simulink model "cmtdtool_sampleharness"  (Simulink 7.1)
settings: Solver=FixedStepDiscrete  StartTime=0.0  StopTime=10.0  FixedStep=0.01  RelTol=1e-3
undefined symbols (not defined in the file or in its folder): DiscIntNeverNeededParam, sigbuilder_block
libraries: simulink x2
settings Model: SldvGeneratedHarnessModel=TestUnitModel=cmtdtool_samplemode|  Creator=The MathWorks Inc.  LastModifiedBy=itoy  CovMetricSettings=dcmoe  CovHTMLOptions=-aTS=1 -bRG=1 -bTC=0 -hTR=0 -nFC=0 -scm=1 -bcm=1 -xEv=0  covSaveCumulativeToWorkspaceVar=off  CovSaveSingleToWorkspaceVar=off  CovModelRefEnable=off
settings OptimizationCC: ConditionallyExecuteInputs=off  InlineParams=on  InlineInvariantSignals=on
settings DebuggingCC: SaveWithParameterizedLinksMsg=none  SignalResolutionControl=TryResolveAllWithWarning  InheritedTsInSrcMsg=none
settings GRTTargetCC: TargetFcnLib=ansi_tfl_tmw.mat  CPPClassGenCompliant=off
settings ConfigComp: Description=Design Verifier Custom Configuration Component  DVMaxProcessTime=60  DVDisplayUnsatisfiableObjectives=on  DVAutomaticStubbing=off  DVMakeOutputFilesUnique=off  DVParameters=on  DVModelCoverageObjectives=MCDC  DVMaxTestCaseSteps=500  DVTestSuiteOptimization=CombinedObjectives  DVAssertions=EnableAll  DVProofAssumptions=EnableAll  DVProvingStrategy=FindViolation  DVSaveHarnessModel=on  DVSaveReport=on

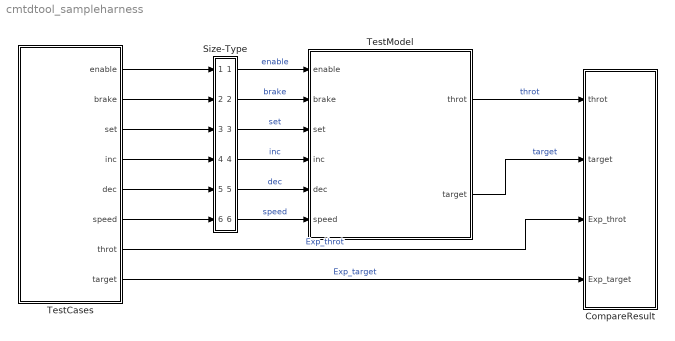
== system cmtdtool_sampleharness ==
  CompareResult : Subsystem  DisableCoverage=on
  Size-Type : Subsystem
  TestCases : Subsystem  Tag=STV Subsys  LoadFcn=sigbuilder_block('load',[49.5 50.25 519.75 399.75 ]);  StartFcn=sigbuilder_block('start');  StopFcn=sigbuilder_block('stop');  ClipboardFcn=sigbuilder_block('clipboard');  mask(Sigbuilder block){}
      mask init:
      | if ~strcmp(get_param(bdroot(gcb),'SimulationStatus'),'stopped') tuvar = sigbuilder_block('maskInit'); end
      settings: CopyFcn=sigbuilder_block('copy');  DeleteFcn=sigbuilder_block('delete');  ModelCloseFcn=sigbuilder_block('modelClose');  PreSaveFcn=sigbuilder_block('preSave');  NameChangeFcn=sigbuilder_block('namechange');  OpenFcn=sigbuilder_block('open');  CloseFcn=sigbuilder_block('close');
      mask Display: plot(0,0,100,100,[10,10,40,40,10],[80,20,20,80,80],[40,10],[50,50], [40,27,10],[65,72,56],[40,25,25,10],[28,28,43,43]);
  TestModel : Subsystem
  wires:
  Size-Type/1(Out1) -> TestModel/1(enable)  "enable"
  Size-Type/2(Out2) -> TestModel/2(brake)  "brake"
  Size-Type/3(Out3) -> TestModel/3(set)  "set"
  Size-Type/4(Out4) -> TestModel/4(inc)  "inc"
  Size-Type/5(Out5) -> TestModel/5(dec)  "dec"
  Size-Type/6(Out6) -> TestModel/6(speed)  "speed"
  TestCases/1(enable) -> Size-Type/1(In1)
  TestCases/2(brake) -> Size-Type/2(In2)
  TestCases/3(set) -> Size-Type/3(In3)
  TestCases/4(inc) -> Size-Type/4(In4)
  TestCases/5(dec) -> Size-Type/5(In5)
  TestCases/6(speed) -> Size-Type/6(In6)
  TestModel/1(throt) -> CompareResult/1(throt)  "throt"
  TestCases/7(throt) -> CompareResult/3(Exp_throt)  "Exp_throt"
  TestModel/2(target) -> CompareResult/2(target)  "target"
  TestCases/8(target) -> CompareResult/4(Exp_target)  "Exp_target"

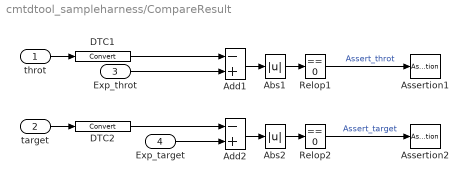
== system cmtdtool_sampleharness/CompareResult ==
  throt : Inport
  target : Inport  Port=2
  Exp_throt : Inport  Port=3
  Exp_target : Inport  Port=4
  Abs1 : Abs  SaturateOnIntegerOverflow=on
  Abs2 : Abs  SaturateOnIntegerOverflow=on
  Add1 : Sum  Inputs=-+  AccumDataTypeStr=double  OutDataTypeStr=double  SaturateOnIntegerOverflow=on  InputSameDT=on
  Add2 : Sum  Inputs=-+  AccumDataTypeStr=double  OutDataTypeStr=double  SaturateOnIntegerOverflow=on  InputSameDT=on
  Assertion1 : Assertion  Enabled=on  StopWhenAssertionFail=off
  Assertion2 : Assertion  Enabled=on  StopWhenAssertionFail=off
  DTC1 : DataTypeConversion
  DTC2 : DataTypeConversion
  Relop1 : simulink/Logic and Bit Operations/Compare To Constant  SystemSampleTime=-1  relop===  const=0  LogicOutDataTypeMode=uint8
  Relop2 : simulink/Logic and Bit Operations/Compare To Constant  SystemSampleTime=-1  relop===  const=0  LogicOutDataTypeMode=uint8
  wires:
  DTC1/1 -> Add1/1
  Add1/1 -> Abs1/1
  Abs1/1 -> Relop1/1
  Relop1/1 -> Assertion1/1  "Assert_throt"
  DTC2/1 -> Add2/1
  Add2/1 -> Abs2/1
  Abs2/1 -> Relop2/1
  Relop2/1 -> Assertion2/1  "Assert_target"
  throt/1 -> DTC1/1
  Exp_throt/1 -> Add1/2
  target/1 -> DTC2/1
  Exp_target/1 -> Add2/2

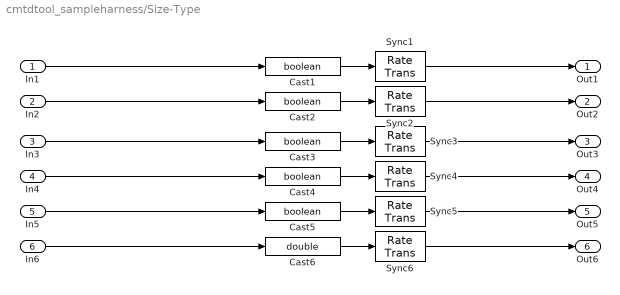
== system cmtdtool_sampleharness/Size-Type ==
  In1 : Inport
  In2 : Inport  Port=2
  In3 : Inport  Port=3
  In4 : Inport  Port=4
  In5 : Inport  Port=5
  In6 : Inport  Port=6
  Cast{1..5} (5 alike) : DataTypeConversion  OutDataTypeStr=boolean  SaturateOnIntegerOverflow=on  RndMeth=Zero
  Cast6 : DataTypeConversion  OutDataTypeStr=double  SaturateOnIntegerOverflow=on  RndMeth=Zero
  Sync{1..6} (6 alike) : RateTransition  OutPortSampleTime=[0.01,0]
  Out1 : Outport
  Out2 : Outport  Port=2
  Out3 : Outport  Port=3
  Out4 : Outport  Port=4
  Out5 : Outport  Port=5
  Out6 : Outport  Port=6
  wires:
  In1/1 -> Cast1/1
  Cast1/1 -> Sync1/1
  Sync1/1 -> Out1/1
  In2/1 -> Cast2/1
  Cast2/1 -> Sync2/1
  Sync2/1 -> Out2/1
  In3/1 -> Cast3/1
  Cast3/1 -> Sync3/1
  Sync3/1 -> Out3/1
  In4/1 -> Cast4/1
  Cast4/1 -> Sync4/1
  Sync4/1 -> Out4/1
  In5/1 -> Cast5/1
  Cast5/1 -> Sync5/1
  Sync5/1 -> Out5/1
  In6/1 -> Cast6/1
  Cast6/1 -> Sync6/1
  Sync6/1 -> Out6/1

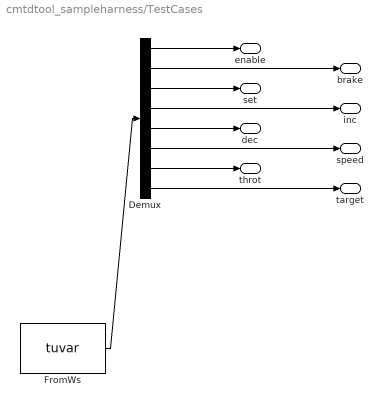
== system cmtdtool_sampleharness/TestCases ==
  Demux : Demux  Tag=STV Demux  Outputs=8
  FromWs : FromWorkspace  Tag=STV FromWs  VariableName=tuvar  SampleTime=0  SigBuilderData=DataTag0  VnvData=DataTag1
      SigBuilderData=|
      | channels(1).label = 'enable'
      | channels(1).allXData = {[0 0.01 0.02 0.03 0.04 0.05 0.06 0.07 0.08 0.09 0.1 0.11], [0 0.01 0.02 0.03 0.04 0.05 0.06 0.07 0.08 0.09 0.1 0.11], [0 0.01 0.02 0.03 0.04 0.05 0.06 0.07 0.08 0.09 0.1 0.11], [0 0.01 0.02 0.03 0.04 0.05 0.06 0.07 0.08 0.09 0.1 0.11], [0 0.01 0.02 0.03 0.04 0.05 0.06 0.07 0.08 0.09 0.1 0.11 0.12]}
      | channels(1).allYData = {[1 1 1 1 1 1 1 1 1 1 1 1], [1 1 1 1 1 1 1 1 1 1 1 1], [1 1 1 1 1 1 1 1 1 1 1 1], [0 0 0 0 0 0 0 0 0 0 0 0], [0 0 0 0 0 0 0 0 0 0 0 0 0]}
      | channels(2).label = 'brake'
      | channels(2).allXData = {[0 0.01 0.02 0.03 0.03 0.04 0.05 0.06 0.07 0.08 0.09 0.1 0.11], [0 0.01 0.02 0.03 0.04 0.05 0.06 0.07 0.08 0.09 0.1 0.11], [0 0.01 0.01 0.02 0.03 0.04 0.05 0.06 0.07 0.08 0.09 0.1 0.11], [0 0.01 0.02 0.03 0.04 0.05 0.06 0.07 0.08 0.09 0.1 0.11], [0 0.01 0.02 0.03 0.04 0.05 0.06 0.07 0.08 0.09 0.1 0.11 0.12]}
      | channels(2).allYData = {[1 1 1 1 0 0 0 0 0 0 0 0 0], [0 0 0 0 0 0 0 0 0 0 0 0], [0 0 1 1 1 1 1 1 1 1 1 1 1], [0 0 0 0 0 0 0 0 0 0 0 0], [0 0 0 0 0 0 0 0 0 0 0 0 0]}
      | channels(3).label = 'set'
      | channels(3).allXData = {[0 0.01 0.02 0.03 0.04 0.04 0.05 0.06 0.07 0.08 0.09 0.1 0.1 0.11], [0 0.01 0.01 0.02 0.03 0.04 0.05 0.06 0.07 0.08 0.09 0.1 0.11], [0 0.01 0.01 0.02 0.03 0.04 0.05 0.06 0.07 0.08 0.09 0.1 0.11], [0 0.01 0.02 0.03 0.04 0.05 0.06 0.07 0.08 0.09 0.1 0.11], [0 0.01 0.02 0.03 0.04 0.05 0.06 0.07 0.08 0.09 0.1 0.11 0.12]}
      | channels(3).allYData = {[1 1 1 1 1 0 0 0 0 0 0 0 1 1], [1 1 0 0 0 0 0 0 0 0 0 0 0], [1 1 0 0 0 0 0 0 0 0 0 0 0], [0 0 0 0 0 0 0 0 0 0 0 0], [0 0 0 0 0 0 0 0 0 0 0 0 0]}
      | channels(4).label = 'inc'
      | channels(4).allXData = {[0 0.01 0.02 0.03 0.04 0.05 0.06 0.07 0.08 0.09 0.09 0.1 0.11], [0 0.01 0.01 0.02 0.03 0.04 0.05 0.06 0.07 0.08 0.09 0.1 0.11], [0 0.01 0.01 0.02 0.03 0.04 0.05 0.06 0.07 0.08 0.09 0.1 0.11], [0 0.01 0.02 0.03 0.04 0.05 0.06 0.07 0.08 0.09 0.1 0.11], [0 0.01 0.02 0.03 0.04 0.05 0.06 0.07 0.08 0.09 0.1 0.11 0.12]}
      | channels(4).allYData = {[1 1 1 1 1 1 1 1 1 1 0 0 0], [1 1 0 0 0 0 0 0 0 0 0 0 0], [1 1 0 0 0 0 0 0 0 0 0 0 0], [0 0 0 0 0 0 0 0 0 0 0 0], [0 0 0 0 0 0 0 0 0 0 0 0 0]}
      | channels(5).label = 'dec'
      | channels(5).allXData = {[0 0.01 0.02 0.03 0.04 0.05 0.06 0.07 0.08 0.09 0.1 0.11], [0 0.01 0.01 0.02 0.03 0.04 0.05 0.06 0.07 0.07 0.08 0.09 0.1 0.11], [0 0.01 0.02 0.03 0.04 0.05 0.06 0.07 0.08 0.09 0.1 0.11], [0 0.01 0.02 0.03 0.04 0.05 0.06 0.07 0.08 0.09 0.1 0.11], [0 0.01 0.02 0.03 0.04 0.05 0.06 0.07 0.08 0.09 0.1 0.11 0.12]}
      | channels(5).allYData = {[0 0 0 0 0 0 0 0 0 0 0 0], [0 0 1 1 1 1 1 1 1 0 0 0 0 0], [0 0 0 0 0 0 0 0 0 0 0 0], [0 0 0 0 0 0 0 0 0 0 0 0], [1 1 1 1 1 1 1 1 1 1 1 1 1]}
      | channels(6).label = 'speed'
      | channels(6).allXData = {[0 0.01 0.01 0.02 0.02 0.03 0.03 0.04 0.04 0.05 0.05 0.06 0.06 0.07 0.08 0.09 0.1 0.1 0.11], [0 0.01 0.01 0.02 0.02 0.03 0.04 0.04 0.05 0.05 0.06 0.07 0.07 0.08 0.09 0.1 0.11], [0 0.01 0.01 0.02 0.03 0.04 0.05 0.06 0.07 0.08 0.09 0.1 0.11], [0 0.01 0.02 0.03 0.04 0.05 0.06 0.07 0.08 0.09 0.1 0.11], [0 0.01 0.02 0.03 0.04 0.05 0.06 0.07 0.08 0.09 0.1 0.11 0.12]}
      | channels(6).allYData = {[0 0 30 30 60 60 90 90 50 50 10 10 0 0 0 0 0 30 30], [0 0 30 30 60 60 60 90 90 120 120 120 80 80 80 80 80], [0 0 30 30 30 30 30 30 30 30 30 30 30], [0 0 0 0 0 0 0 0 0 0 0 0], [0 0 0 0 0 0 0 0 0 0 0 0 0]}
      | channels(7).label = 'throt'
      | channels(7).allXData = {[0 0.01 0.02 0.03 0.04 0.04 0.05 0.05 0.06 0.06 0.07 0.07 0.08 0.08 0.09 0.09 0.1 0.1 0.11], [0 0.01 0.01 0.02 0.02 0.03 0.03 0.04 0.04 0.05 0.05 0.06 0.06 0.07 0.07 0.08 0.09 0.1 0.11], [0 0.01 0.02 0.03 0.04 0.05 0.06 0.07 0.08 0.09 0.1 0.11], [0 0.01 0.02 0.03 0.04 0.05 0.06 0.07 0.08 0.09 0.1 0.11], [0 0.01 0.02 0.03 0.04 0.05 0.06 0.07 0.08 0.09 0.1 0.11 0.12]}
      | channels(7).allYData = {[0 0 0 0 0 0.82 0.82 1.6441 1.6441 1.8723 1.8723 1.9016 1.9016 1.931 1.931 1.9405 1.9405 0.05 0.05], [0 0 -0.62 -0.62 -1.2431 -1.2431 -1.2693 -1.2693 -1.8956 -1.8956 -2.525 -2.525 -2.5575 -2.5575 -1.77 -1.77 -1.77 -1.77 -1.77], [0 0 0 0 0 0 0 0 0 0 0 0], [0 0 0 0 0 0 0 0 0 0 0 0], [0 0 0 0 0 0 0 0 0 0 0 0 0]}
      | channels(8).label = 'target'
      | channels(8).allXData = {[0 0.01 0.01 0.02 0.02 0.03 0.03 0.04 0.04 0.05 0.05 0.06 0.06 0.07 0.07 0.08 0.08 0.09 0.1 0.1 0.11], [0 0.01 0.01 0.02 0.02 0.03 0.03 0.04 0.04 0.05 0.05 0.06 0.06 0.07 0.08 0.09 0.1 0.11], [0 0.01 0.02 0.03 0.04 0.05 0.06 0.07 0.08 0.09 0.1 0.11], [0 0.01 0.02 0.03 0.04 0.05 0.06 0.07 0.08 0.09 0.1 0.11], [0 0.01 0.01 0.02 0.02 0.03 0.03 0.04 0.04 0.05 0.05 0.06 0.06 0.07 0.07 0.08 0.08 0.09 0.09 0.1 0.1 0.11 0.11 0.12]}
      | channels(8).allYData = {[0 0 30 30 60 60 90 90 91 91 92 92 93 93 94 94 95 95 95 30 30], [0 0 -1 -1 -2 -2 -3 -3 -4 -4 -5 -5 -6 -6 -6 -6 -6 -6], [0 0 0 0 0 0 0 0 0 0 0 0], [0 0 0 0 0 0 0 0 0 0 0 0], [-1 -1 -2 -2 -3 -3 -4 -4 -5 -5 -6 -6 -7 -7 -8 -8 -9 -9 -10 -10 -11 -11 -12 -12]}
      | dataSet(1).timeRange = [0 0.11]
      | dataSet(1).name = 'Test Case 01'
      | dataSet(2).timeRange = [0 0.11]
      | dataSet(2).name = 'Test Case 02'
      | dataSet(3).timeRange = [0 0.11]
      | dataSet(3).name = 'Test Case 03'
      | dataSet(4).timeRange = [0 0.11]
      | dataSet(4).name = 'Test Case 04'
      | dataSet(5).timeRange = [0 0.12]
      | dataSet(5).name = 'Test Case 05'
  enable : Outport  Tag=STV Outport
  brake : Outport  Tag=STV Outport  Port=2
  set : Outport  Tag=STV Outport  Port=3
  inc : Outport  Tag=STV Outport  Port=4
  dec : Outport  Tag=STV Outport  Port=5
  speed : Outport  Tag=STV Outport  Port=6
  throt : Outport  Tag=STV Outport  Port=7
  target : Outport  Tag=STV Outport  Port=8
  wires:
  Demux/8 -> target/1
  Demux/7 -> throt/1
  Demux/6 -> speed/1
  Demux/5 -> dec/1
  Demux/4 -> inc/1
  Demux/3 -> set/1
  Demux/2 -> brake/1
  Demux/1 -> enable/1
  FromWs/1 -> Demux/1

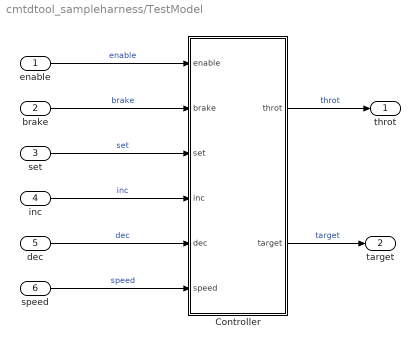
== system cmtdtool_sampleharness/TestModel ==
  enable : Inport  OutDataTypeStr=boolean
  brake : Inport  Port=2  OutDataTypeStr=boolean
  set : Inport  Port=3  OutDataTypeStr=boolean
  inc : Inport  Port=4  OutDataTypeStr=boolean
  dec : Inport  Port=5  OutDataTypeStr=boolean
  speed : Inport  Port=6  OutDataTypeStr=double
  Controller : Subsystem
  throt : Outport
  target : Outport  Port=2
  wires:
  speed/1 -> Controller/6(speed)  "speed"
  Controller/2(target) -> target/1  "target"
  dec/1 -> Controller/5(dec)  "dec"
  inc/1 -> Controller/4(inc)  "inc"
  Controller/1(throt) -> throt/1  "throt"
  set/1 -> Controller/3(set)  "set"
  brake/1 -> Controller/2(brake)  "brake"
  enable/1 -> Controller/1(enable)  "enable"

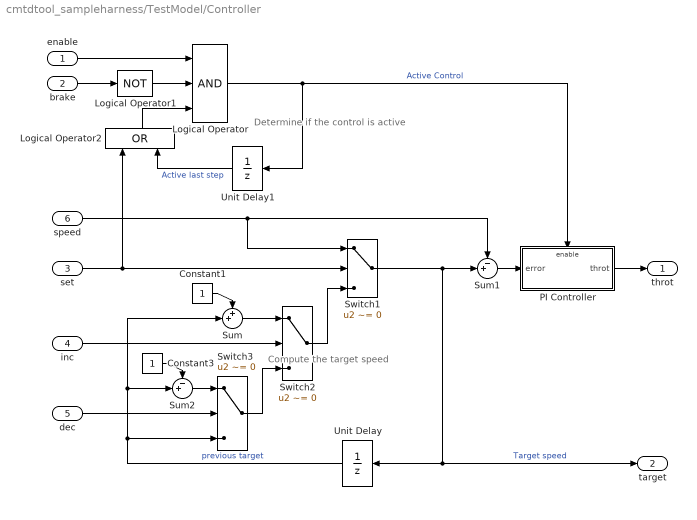
== system cmtdtool_sampleharness/TestModel/Controller ==
  note: Compute the
      | target speed
  note: Determine if the
      | control is active
  enable : Inport  OutDataTypeStr=boolean
  brake : Inport  Port=2  OutDataTypeStr=boolean
  set : Inport  Port=3  OutDataTypeStr=boolean
  inc : Inport  Port=4  OutDataTypeStr=boolean
  dec : Inport  Port=5  OutDataTypeStr=boolean
  speed : Inport  Port=6  OutDataTypeStr=double
  Constant1 : Constant
  Constant3 : Constant
  Logical Operator : Logic  Inputs=3  AllPortsSameDT=off  OutDataTypeStr=boolean
  Logical Operator1 : Logic  Operator=NOT  AllPortsSameDT=off  OutDataTypeStr=boolean
  Logical Operator2 : Logic  Orientation=up  Operator=OR  AllPortsSameDT=off  OutDataTypeStr=boolean
  PI Controller : Subsystem
  Sum : Sum  Inputs=++|
  Sum1 : Sum  Inputs=-+|
  Sum2 : Sum  Inputs=-+|
  Switch1 : Switch  Criteria=u2 ~= 0
  Switch2 : Switch  Criteria=u2 ~= 0
  Switch3 : Switch  Criteria=u2 ~= 0
  Unit Delay : UnitDelay  Orientation=left  SampleTime=0.01
  Unit Delay1 : UnitDelay  Orientation=left  SampleTime=0.01
  throt : Outport
  target : Outport  Port=2
  wires:
  PI Controller/1(throt) -> throt/1
  Sum1/1 -> PI Controller/1(error)
  Logical Operator/1 -> PI Controller/Enable, Unit Delay1/1  "Active Control"
  Unit Delay1/1 -> Logical Operator2/2  "Active last step"
  Logical Operator2/1 -> Logical Operator/3
  Switch1/1 -> Sum1/2, target/1, Unit Delay/1  "Target speed"
  Unit Delay/1 -> Switch3/3, Sum2/2, Sum/2  "previous target"
  Switch3/1 -> Switch2/3
  Switch2/1 -> Switch1/3
  Sum2/1 -> Switch3/1
  Constant3/1 -> Sum2/1
  dec/1 -> Switch3/2
  Sum/1 -> Switch2/1
  Constant1/1 -> Sum/1
  inc/1 -> Switch2/2
  speed/1 -> Switch1/1, Sum1/1
  set/1 -> Logical Operator2/1, Switch1/2
  Logical Operator1/1 -> Logical Operator/2
  enable/1 -> Logical Operator/1
  brake/1 -> Logical Operator1/1

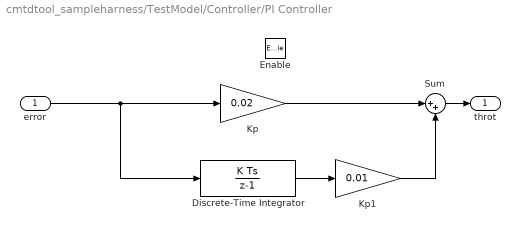
== system cmtdtool_sampleharness/TestModel/Controller/PI Controller ==
  error : Inport
  Enable : EnablePort
  Discrete-Time Integrator : DiscreteIntegrator  SampleTime=0.01  LimitOutput=on  UpperSaturationLimit=5  LowerSaturationLimit=-5  ICPrevOutput=DiscIntNeverNeededParam  ICPrevScaledInput=DiscIntNeverNeededParam
  Kp : Gain  Gain=0.02
  Kp1 : Gain  Gain=0.01
  Sum : Sum  Inputs=|++
  throt : Outport
  wires:
  Sum/1 -> throt/1
  error/1 -> Discrete-Time Integrator/1, Kp/1
  Discrete-Time Integrator/1 -> Kp1/1
  Kp1/1 -> Sum/2
  Kp/1 -> Sum/1
